simulink model "Model"  (R2023b)
settings: Solver=ode4  StartTime=0.0  StopTime=7.121081656184960e+03  FixedStep=0.1  RelTol=1e-3
values from neighbouring files (symbols this model uses):
  astro_data = astronomicData    [main.m]
  in_cond = initialConditions(astro_data.n_eth)    [main.m]
  orbit_data = orbitData    [main.m]
  pert_data = perturbationData(orbit_data.n_sc)    [main.m]
  sc_data = spaceCraftData    [main.m]
undefined symbols (not defined in the file or in its folder): A_target, k1, k2, Kdx, Kdy, Kdz, Kpx, Kpy, Kpz, sensor_data
libraries: matrix_library x6, simulink x5, vrlib x4
(part 1 of 2)
settings Model: Creator=pierb  LastModifiedBy=pierb

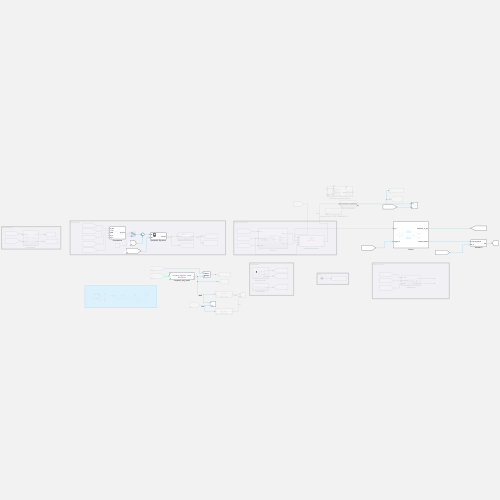
[thumbnail: Simulink's stored preview of the top-level diagram]
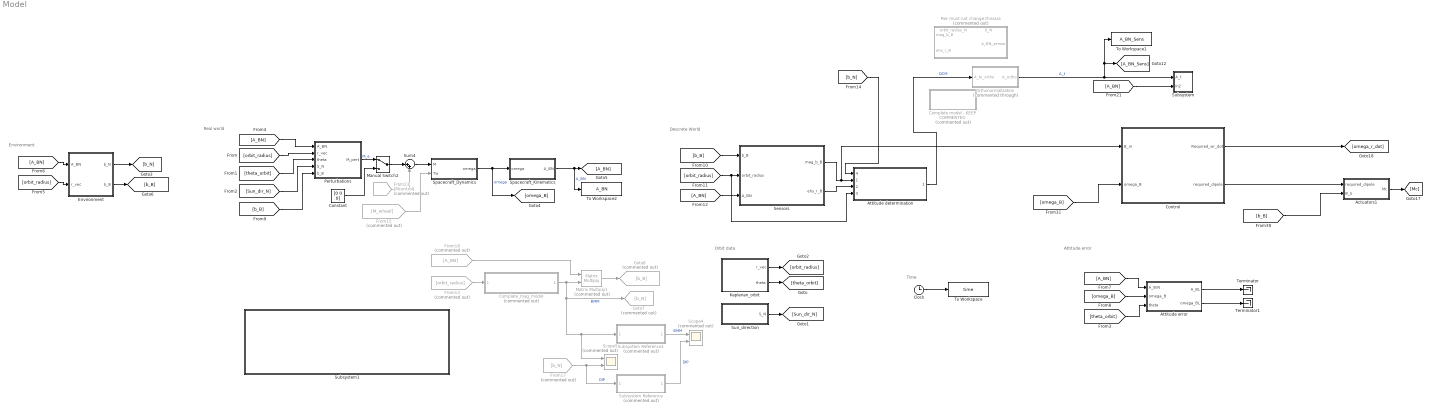
== system Model ==
  note: Descrete World
  note: Environment
  note: Attitude error
  note: Real world
  note: Orbit data
  note: Time
  Actuators1 : Subsystem
  Attitude determination : Subsystem  ReferencedSubsystem=TRIAD
      settings: PortSchema="{\"entries\":[{\"content\":{\"sides\":[{\"content\":{\"connectorIds\":[\"In4\",\"In1\",\"In2\",\"In3\"]},\"type\":\"ConnectorPlacement.EquallySpacedRectSide\",\"uuid\":\"0502630d-a8df-43ec-b57f-23f371792df2\"},{\"content\":{\"connectorIds\":[\"Out1\"],\"side\":\"RIGHT\"},\"type\":\"ConnectorPlacement.EquallySpacedRectSide\",\"uuid\":\"e2538cd4-94c7-4835-89c8-02f932021d19\"},{\"content\":{\"side\":\"TOP\"},\"type\":\"ConnectorPlacement.EquallySpacedRectSide\",\"uuid\":\"052200ab-1f19-47f5-82ad-2a8e946d4726\"},{\"content\":{\"side\":\"BOTTOM\"},\"type\":\"ConnectorPlacement.EquallySpacedRectSide\",\"uuid\":\"8f6caf11-bde2-49b2-b877-be2d81d96931\"}]},\"type\":\"ConnectorPlacement.EquallySpacedConnector\",\"uuid\":\"0adaba7c-309a-4af6-b194-7fbfafdbd17f\"}],\"packageUris\":[\"http://schema.mathworks.com/mf0/Connector/R2020b\"],\"version\":\"1.0\"}"
  Attitude error : Subsystem
  Clock : Clock
  Complete model - KEEP COMMENTED : Subsystem  Commented=on
  Complete_mag_model : Subsystem  Commented=on  ReferencedSubsystem=complete_magnetic_model
  Constant : Constant  Value=[0 0 0]
  Control : Subsystem
  Environment : Subsystem
  From13 : From  Commented=on  GotoTag=orbit_radius
  From15 : From  Commented=on  GotoTag=M_wheel
  From17 : From  Commented=on  GotoTag=b_N
  From18 : From  Commented=on  GotoTag=A_BN
  From23 : From  Commented=on  GotoTag=Mcontrol
  Goto7 : Goto  Commented=on  GotoTag=b_N
  Goto8 : Goto  Commented=on  GotoTag=b_B
  Keplerian_orbit : Subsystem
  Manual Switch2 : ManualSwitch
  Matrix Multiply1 : Product  Commented=on  Multiplication=Matrix(*)
  Orthonormalization : Subsystem  Commented=through
  Perturbations : Subsystem
  Pier must not change thisssss : Subsystem  Commented=on
      settings: PortSchema="{\"entries\":[{\"content\":{\"sides\":[{\"content\":{\"connectorIds\":[\"In1\",\"In2\"]},\"type\":\"ConnectorPlacement.EquallySpacedRectSide\",\"uuid\":\"0502630d-a8df-43ec-b57f-23f371792df2\"},{\"content\":{\"connectorIds\":[\"Out1\"],\"side\":\"RIGHT\"},\"type\":\"ConnectorPlacement.EquallySpacedRectSide\",\"uuid\":\"e2538cd4-94c7-4835-89c8-02f932021d19\"},{\"content\":{\"connectorIds\":[\"In3\",\"In4\"],\"side\":\"TOP\"},\"type\":\"ConnectorPlacement.EquallySpacedRectSide\",\"uuid\":\"052200ab-1f19-47f5-82ad-2a8e946d4726\"}]},\"type\":\"ConnectorPlacement.EquallySpacedConnector\",\"uuid\":\"0adaba7c-309a-4af6-b194-7fbfafdbd17f\"}],\"packageUris\":[\"http://schema.mathworks.com/mf0/Connector/R2020b\"],\"version\":\"1.0\"}"
  Scope4 : Scope  Commented=on  NumInputPorts=2
  Scope5 : Scope  Commented=on  NumInputPorts=2
  Sensors : Subsystem
  Spacecraft_Dynamics : Subsystem
  Spacecraft_Kinematics : Subsystem
  Subsystem : Subsystem
  Subsystem Reference : Subsystem  Commented=on  ReferencedSubsystem=vec_norm
  Subsystem Reference1 : Subsystem  Commented=on  ReferencedSubsystem=vec_norm
  Subsystem1 : Subsystem
  Sum4 : Sum  Inputs=|++
  Sun_direction : Subsystem
  Terminator : Terminator
  Terminator1 : Terminator
  To Workspace : ToWorkspace  VariableName=time  SampleTime=-1
      settings: Save2DSignal=2-D array (concatenate along first dimension)
  To Workspace1 : ToWorkspace  VariableName=A_BN_Sens  SampleTime=-1
  To Workspace2 : ToWorkspace  VariableName=A_BN  SampleTime=-1
  wires:
  Spacecraft_Dynamics/1(omega) -> [omega_B], Spacecraft_Kinematics/1(omega)  "omega"
  Spacecraft_Kinematics/1(A_BN) -> To Workspace2/1, [A_BN]  "A_BN"
  Clock/1 -> To Workspace/1
  Perturbations/1(M_pert) -> Manual Switch2/1  "M_e"
  Manual Switch2/1 -> Sum4/1
  Constant/1 -> Manual Switch2/2
  Attitude error/2(omega_BL) -> Terminator1/1
  Attitude error/1(A_BL) -> Terminator/1
  Keplerian_orbit/2(theta) -> [theta_orbit]
  Sun_direction/1(S_N) -> [Sun_dir_N]
  [orbit_radius] -> Perturbations/2(r_vec)
  [theta_orbit] -> Perturbations/3(theta)
  [Sun_dir_N] -> Perturbations/4(S_N)
  [theta_orbit] -> Attitude error/3(theta)
  [A_BN] -> Perturbations/1(A_BN)
  [A_BN] -> Attitude error/1(A_B/N)
  [omega_B] -> Attitude error/2(omega_B)
  Keplerian_orbit/1(r_vec) -> [orbit_radius]
  [orbit_radius] -> Environment/2(r_vec)
  [A_BN] -> Environment/1(A_BN)
  Environment/2(b_B) -> [b_B]
  Environment/1(b_N) -> [b_N]
  [b_B] -> Perturbations/5(b_B)
  [b_B] -> Sensors/1(b_B)
  [orbit_radius] -> Attitude determination/3, Sensors/2(orbit_radius)
  Sensors/2(ehs_r_B) -> Attitude determination/2
  Attitude determination/1 -> Orthonormalization/1(A_to_ortho)  "DCM"
  [b_N] -> Attitude determination/4
  [A_BN] -> Sensors/3(A_BN)
  Subsystem Reference1/1 -> Scope4/1  "BMM"
  Matrix Multiply1/1 -> Goto8/1
  From18/1 -> Matrix Multiply1/1
  From17/1 -> Subsystem Reference/1, Scope5/2  "DIP"
  Complete_mag_model/1 -> Matrix Multiply1/2, Subsystem Reference1/1, Scope5/1, Goto7/1  "BMM"
  Subsystem Reference/1 -> Scope4/2  "DIP"
  From13/1 -> Complete_mag_model/1
  Sum4/1 -> Spacecraft_Dynamics/1(M)
  From23/1 -> Sum4/2
  From15/1 -> Spacecraft_Dynamics/2(Tw)
  Orthonormalization/1(A_ortho) -> To Workspace1/1, [A_BN_Sens], Subsystem/1(A_t)  "A_t"
  [A_BN] -> Subsystem/2(In2)
  Control/1(Required_wr_dot) -> [omega_r_dot]
  Control/2(required_dipole) -> Actuators1/1(required_dipole)
  [omega_B] -> Control/2(omega_B)
  Actuators1/1(Mc) -> [Mc]
  Sensors/1(mag_b_B) -> Attitude determination/1, Control/1(B_m)
  [b_B] -> Actuators1/2(B_b)

== system Model/Actuators1 ==
  required_dipole : Inport
  B_b : Inport  Port=2
  Apply_inertia : Subsystem
  Cross Product : matrix_library/Cross Product
  Reshape : Reshape  OutputDimensionality=Row vector (2-D)
  Saturation : Saturate  UpperLimit=120  LowerLimit=-120
  Mc : Outport
  wires:
  required_dipole/1 -> Saturation/1
  Saturation/1 -> Cross Product/1
  B_b/1 -> Cross Product/2
  Apply_inertia/1(Torque_omega_dot) -> Mc/1  "I^-1 * M"
  Reshape/1 -> Apply_inertia/1(M)
  Cross Product/1 -> Reshape/1

== system Model/Attitude error ==
  A_B/N : Inport
  omega_B : Inport  Port=2
  theta : Inport  Port=3
  A_LN : Subsystem
  Add : Sum  Inputs=-+
  Constant : Constant  Value=pert_data.w_LN
  Product : Product  Multiplication=Matrix(*)
  Product1 : Product  Multiplication=Matrix(*)
  Reshape : Reshape  OutputDimensionality=Column vector (2-D)
  Reshape1 : Reshape  OutputDimensionality=Column vector (2-D)
  Reshape2 : Reshape  OutputDimensionality=Row vector (2-D)
  To Workspace2 : ToWorkspace  VariableName=w_BL  SampleTime=-1
      settings: Save2DSignal=2-D array (concatenate along first dimension)
  Transpose : Math  Operator=transpose
  A_BL : Outport
  omega_BL : Outport  Port=2
  wires:
  A_LN/1(A_LN) -> Transpose/1
  Transpose/1 -> Product/2
  A_B/N/1 -> Product/1
  Product/1 -> Product1/1, A_BL/1
  omega_B/1 -> Reshape1/1
  Constant/1 -> Reshape/1
  Product1/1 -> Add/1
  Reshape/1 -> Product1/2
  Reshape1/1 -> Add/2
  theta/1 -> A_LN/1(theta)
  Add/1 -> Reshape2/1
  Reshape2/1 -> To Workspace2/1, omega_BL/1

== system Model/Complete model - KEEP COMMENTED ==
  Actuators : Subsystem  Commented=on
  Attitude determination : Subsystem  Commented=on
  Control : Subsystem  Commented=on
  Environment : Subsystem  Commented=on
  Perturbations1 : Subsystem  Commented=on
  Scope1 : Scope  Commented=on
  Sensors : Subsystem  Commented=on
      settings: PortSchema="{\"entries\":[{\"content\":{\"sides\":[{\"content\":{\"connectorIds\":[\"In1\"]},\"type\":\"ConnectorPlacement.EquallySpacedRectSide\",\"uuid\":\"59271294-fd38-4bc9-bb13-2c1f308ccf3d\"},{\"content\":{\"connectorIds\":[\"Out1\"],\"side\":\"RIGHT\"},\"type\":\"ConnectorPlacement.EquallySpacedRectSide\",\"uuid\":\"0ccf848c-1fca-40cd-9aef-56cdc22c78d6\"},{\"content\":{\"connectorIds\":[\"In2\"],\"side\":\"TOP\"},\"type\":\"ConnectorPlacement.EquallySpacedRectSide\",\"uuid\":\"ccb51de9-ba45-4790-8cdc-dbedbef5dfe7\"}]},\"type\":\"ConnectorPlacement.EquallySpacedConnector\",\"uuid\":\"d2012a93-3259-48d9-8262-2c73c3498720\"}],\"packageUris\":[\"http://schema.mathworks.com/mf0/Connector/R2020b\"],\"version\":\"1.0\"}"
  Spacecraft_Dynamics1 : Subsystem  Commented=on
  Spacecraft_Kinematics1 : Subsystem  Commented=on
  Sum : Sum  Commented=on  Inputs=|++
  To Workspace1 : ToWorkspace  Commented=on  VariableName=r_int  SampleTime=-1
      settings: Save2DSignal=2-D array (concatenate along first dimension)
  r_integration : Subsystem  Commented=on
  wires:
  Control/1(Out1) -> Actuators/1(1)
  Actuators/1(Out1) -> Sum/2
  Environment/1(envData) -> Attitude determination/2(envData), Sensors/2(envData)  "envData"
  Perturbations1/1(M_e) -> Sum/1  "M_e"
  Attitude determination/1(A_M) -> Control/1(A_M)  "A_M"
  r_integration/1(r_vec) -> To Workspace1/1, Scope1/1
  Spacecraft_Kinematics1/1(A_T) -> Sensors/1(A_T)  "A_T"
  Sum/1 -> Spacecraft_Dynamics1/1(M)  "M"
  Spacecraft_Dynamics1/1(omega) -> Spacecraft_Kinematics1/1(omega)  "omega"
  Sensors/1(sensorData) -> Attitude determination/1(sensorData)  "sensorData"

== system Model/Control ==
  B_m : Inport
  omega_B : Inport  Port=2
  De-tumbling : Subsystem  TreatAsAtomicUnit=on
  Merge : Merge  Inputs=3  InitialOutput=0
  Merge2 : Merge  Inputs=3  InitialOutput=0
  No control : Subsystem  TreatAsAtomicUnit=on
  Pointing : Subsystem  TreatAsAtomicUnit=on
  String Compare : StringCompare  CaseSensitive=off
  String Compare1 : StringCompare  CaseSensitive=off
  String Constant : StringConstant  String=algorithm
  String Constant1 : StringConstant  String="\"De-tumbling\""
  String Constant2 : StringConstant  String="\"Pointing\""
  XOR : Logic  Operator=NOR  IconShape=distinctive  AllPortsSameDT=off  OutDataTypeStr=boolean
  Required_wr_dot : Outport
  required_dipole : Outport  Port=2
  wires:
  String Constant/1 -> String Compare/2, String Compare1/1
  String Constant1/1 -> String Compare/1
  String Constant2/1 -> String Compare1/2
  String Compare/1 -> De-tumbling/Enable, XOR/1
  String Compare1/1 -> XOR/2, Pointing/Enable
  XOR/1 -> No control/Enable
  De-tumbling/1(Required_wr_dot) -> Merge/1
  No control/1(required_wr_dot) -> Merge/2
  Pointing/1(Required_wr_dot) -> Merge/3
  De-tumbling/2(required_dipole) -> Merge2/1
  No control/2(required_dipole) -> Merge2/2
  Pointing/2(required_dipole) -> Merge2/3
  Merge/1 -> Required_wr_dot/1
  Merge2/1 -> required_dipole/1
  B_m/1 -> De-tumbling/1(B_m)
  omega_B/1 -> De-tumbling/2(omega_B)

== system Model/Environment ==
  A_BN : Inport
  r_vec : Inport  Port=2
  Constant : Constant  Value=astro_data.R_earth
  Constant1 : Constant  Value=pert_data.H0
  Magnetic field : Subsystem  ReferencedSubsystem=dipole_magnetic_model
  Matrix Multiply : Product  Multiplication=Matrix(*)
  Reshape : Reshape  OutputDimensionality=Row vector (2-D)
  Reshape1 : Reshape  OutputDimensionality=Row vector (2-D)
  Subsystem : Subsystem  ReferencedSubsystem=normalize_vec
  Subsystem1 : Subsystem  ReferencedSubsystem=vec_norm
  To Workspace : ToWorkspace  VariableName=env_b_N  SampleTime=-1
      settings: Save2DSignal=2-D array (concatenate along first dimension)
  To Workspace1 : ToWorkspace  VariableName=env_b_B  SampleTime=-1
      settings: Save2DSignal=2-D array (concatenate along first dimension)
  b_N : Outport
  b_B : Outport  Port=2
  wires:
  r_vec/1 -> Subsystem1/1, Subsystem/1
  Reshape/1 -> To Workspace/1
  Reshape1/1 -> To Workspace1/1
  Subsystem/1 -> Magnetic field/1
  Subsystem1/1 -> Magnetic field/2
  Matrix Multiply/1 -> b_B/1, Reshape1/1  "b_B"
  A_BN/1 -> Matrix Multiply/1
  Magnetic field/1 -> Matrix Multiply/2, b_N/1, Reshape/1  "b_N [T]"
  Constant/1 -> Magnetic field/3
  Constant1/1 -> Magnetic field/4

== system Model/Keplerian_orbit ==
  Constant : Constant  Value=in_cond.theta0
  Integrator : Integrator  InitialConditionSource=external  WrapState=on  WrappedStateUpperValue=2*pi  WrappedStateLowerValue=0
  Product : Product
  Reshape : Reshape  OutputDimensionality=Row vector (2-D)
  To Workspace : ToWorkspace  VariableName=kepler_r_vec  SampleTime=-1
      settings: Save2DSignal=2-D array (concatenate along first dimension)
  To Workspace2 : ToWorkspace  VariableName=kepler_theta  SampleTime=-1
      settings: Save2DSignal=2-D array (concatenate along first dimension)
  radius_direction : Subsystem
  radius_mod : Subsystem
  theta_dot : Subsystem
  r_vec : Outport
  theta : Outport  Port=2
  wires:
  theta_dot/1(theta_dot) -> Integrator/1
  Integrator/1 -> theta/1, radius_mod/1(theta), theta_dot/1(theta), radius_direction/1(theta), To Workspace2/1  "theta"
  Constant/1 -> Integrator/2
  radius_direction/1(r_dir) -> Product/1
  radius_mod/1(r_mod) -> Product/2
  Product/1 -> Reshape/1
  Reshape/1 -> To Workspace/1, r_vec/1

== system Model/Orthonormalization ==
  note: $\text{The integration does not preserve the orthonormality of the matrix A, so an iterative method could be implemented. As the error is not high enough to impact substantially the solution, the orthonormalization method is applied only at the first iteration: }\\ A(t) = \frac{3}{2}A_0(t) - \frac{1}{2}A_0(t)A_0^T(t)A_0(t)\\ \text{Note also that this process can be applied only after a certain treshold as been reached to preserve computational power}$
  A_to_ortho : Inport
  Abs : Abs  SaturateOnIntegerOverflow=off
  Constant : Constant  Value=eye(3)
  Constant2 : Constant  Value=1e-6
  If : If  IfExpression=u1 ~= 9
  If Action Subsystem : Subsystem  TreatAsAtomicUnit=on
  If Action Subsystem1 : Subsystem  TreatAsAtomicUnit=on
  Less Than : RelationalOperator  Operator=<=  OutDataTypeStr=boolean  RndMeth=Simplest  InputSameDT=off
  Merge : Merge
  Product1 : Product  Inputs=**  Multiplication=Matrix(*)
  Subtract : Sum  Inputs=+-
  Sum of Elements : Sum  Inputs=+
  Transpose1 : Math  Operator=transpose
  A_ortho : Outport
  wires:
  Product1/1 -> Subtract/1
  Subtract/1 -> Abs/1
  Transpose1/1 -> Product1/2
  Less Than/1 -> Sum of Elements/1
  Constant/1 -> Subtract/2
  Constant2/1 -> Less Than/2
  Abs/1 -> Less Than/1
  Sum of Elements/1 -> If/1
  If/1 -> If Action Subsystem/Action
  If/2 -> If Action Subsystem1/Action
  If Action Subsystem/1(A_ortho) -> Merge/1
  If Action Subsystem1/1(Out1) -> Merge/2
  Merge/1 -> A_ortho/1
  A_to_ortho/1 -> [A_to_ortho]
  [A_to_ortho] -> Product1/1, Transpose1/1
  [A_to_ortho] -> If Action Subsystem1/1(A_to_ortho)
  [A_to_ortho] -> If Action Subsystem/1(A_to_ortho)

== system Model/Perturbations ==
  A_BN : Inport
  r_vec : Inport  Port=2
  theta : Inport  Port=3
  S_N : Inport  Port=4
  b_B : Inport  Port=5
  A_LN : Subsystem
  Add : Sum  Inputs=3
  GG_perturbation : Subsystem  Commented=on
  Magnetic : Subsystem
  SRP : Subsystem  Commented=on
  Subsystem Reference : Subsystem  ReferencedSubsystem=vec_norm
  To Workspace : ToWorkspace  VariableName=perturbations_I_M_GG  SampleTime=-1
      settings: Save2DSignal=2-D array (concatenate along first dimension)
  To Workspace1 : ToWorkspace  VariableName=perturbations_I_M_Mag  SampleTime=-1
      settings: Save2DSignal=2-D array (concatenate along first dimension)
  To Workspace2 : ToWorkspace  VariableName=perturbations_I_M_SRP  SampleTime=-1
      settings: Save2DSignal=2-D array (concatenate along first dimension)
  To Workspace3 : ToWorkspace  VariableName=perturbations_I_M_tot  SampleTime=-1
      settings: Save2DSignal=2-D array (concatenate along first dimension)
  M_pert : Outport
  wires:
  theta/1 -> A_LN/1(theta)
  A_LN/1(A_LN) -> GG_perturbation/1(A_LN)
  A_BN/1 -> SRP/1(A_BN), GG_perturbation/3(A_BN)
  Subsystem Reference/1 -> GG_perturbation/2(r_mod)
  r_vec/1 -> Subsystem Reference/1
  Add/1 -> To Workspace3/1, M_pert/1
  GG_perturbation/1(I_M_GG) -> Add/1, To Workspace/1
  S_N/1 -> SRP/2(S_N)
  Magnetic/1(I_M_Mag) -> To Workspace1/1, Add/3
  SRP/1(I_M_SRP) -> To Workspace2/1, Add/2
  b_B/1 -> Magnetic/1(b_B)

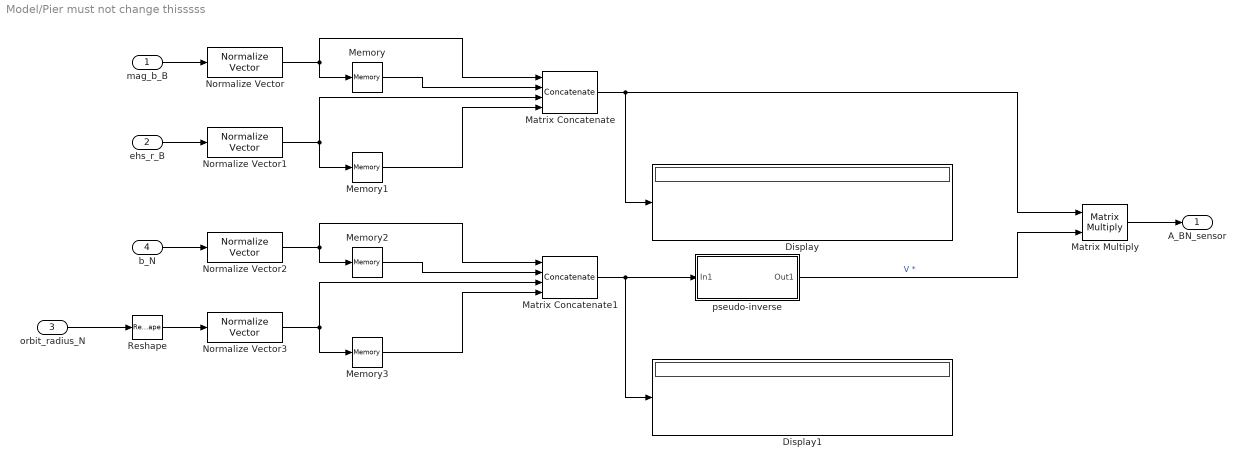
== system Model/Pier must not change thisssss ==
  mag_b_B : Inport
  ehs_r_B : Inport  Port=2
  orbit_radius_N : Inport  Port=3
  b_N : Inport  Port=4
  Display : Display
  Display1 : Display
  Matrix Concatenate : Concatenate  NumInputs=4  Mode=Multidimensional array  ConcatenateDimension=2
  Matrix Concatenate1 : Concatenate  NumInputs=4  Mode=Multidimensional array  ConcatenateDimension=2
  Matrix Multiply : Product  Multiplication=Matrix(*)
  Memory{,1..3} (4 alike) : Memory
  Normalize Vector{,1..3} (4 alike) : vrlib/Utilities/Normalize Vector  maxzero=0
  Reshape : Reshape  OutputDimensionality=Column vector (2-D)
  pseudo-inverse : Subsystem
  A_BN_sensor : Outport
  wires:
  mag_b_B/1 -> Normalize Vector/1
  ehs_r_B/1 -> Normalize Vector1/1
  Matrix Concatenate/1 -> Matrix Multiply/1, Display/1
  Memory/1 -> Matrix Concatenate/2
  Memory1/1 -> Matrix Concatenate/4
  Normalize Vector/1 -> Matrix Concatenate/1, Memory/1
  Normalize Vector1/1 -> Matrix Concatenate/3, Memory1/1
  Normalize Vector2/1 -> Matrix Concatenate1/1, Memory2/1
  Normalize Vector3/1 -> Matrix Concatenate1/3, Memory3/1
  Memory3/1 -> Matrix Concatenate1/4
  b_N/1 -> Normalize Vector2/1
  Memory2/1 -> Matrix Concatenate1/2
  orbit_radius_N/1 -> Reshape/1
  Matrix Concatenate1/1 -> pseudo-inverse/1(In1), Display1/1
  Reshape/1 -> Normalize Vector3/1
  pseudo-inverse/1(Out1) -> Matrix Multiply/2  "V *"
  Matrix Multiply/1 -> A_BN_sensor/1

== system Model/Sensors ==
  b_B : Inport
  orbit_radius : Inport  Port=2
  A_BN : Inport  Port=3
  Digital Clock : DigitalClock  SampleTime=0.1
  Earth horizon sensor : Subsystem  TreatAsAtomicUnit=on  SystemSampleTime=1/sensor_data.magnetometer.freq  ReferencedSubsystem=earth_horizon_sensor
  Magnetometer : Subsystem  SystemSampleTime=1/sensor_data.magnetometer.freq  ReferencedSubsystem=magnetometer_sensor
  Matrix Multiply : Product  Multiplication=Matrix(*)
  Reshape : Reshape  OutputDimensionality=Column vector (2-D)
  Reshape1 : Reshape  OutputDimensionality=Row vector (2-D)
  Reshape2 : Reshape  OutputDimensionality=Row vector (2-D)
  Subsystem Reference : Subsystem  ReferencedSubsystem=normalize_vec
  To Workspace : ToWorkspace  VariableName=sens_magn_B  SampleTime=-1
      settings: Save2DSignal=2-D array (concatenate along first dimension)
  To Workspace1 : ToWorkspace  VariableName=sens_magn_time  SampleTime=-1
      settings: Save2DSignal=2-D array (concatenate along first dimension)
  To Workspace2 : ToWorkspace  VariableName=sens_ehs_r  SampleTime=-1
      settings: Save2DSignal=2-D array (concatenate along first dimension)
  Zero-Order Hold : ZeroOrderHold  SampleTime=1/sensor_data.magnetometer.freq
  Zero-Order Hold1 : ZeroOrderHold  SampleTime=1/sensor_data.horizon.freq
  mag_b_B : Outport
  ehs_r_B : Outport  Port=2
  wires:
  b_B/1 -> Zero-Order Hold/1
  Magnetometer/1 -> mag_b_B/1, Reshape1/1
  Matrix Multiply/1 -> Subsystem Reference/1
  orbit_radius/1 -> Reshape/1
  A_BN/1 -> Matrix Multiply/1
  Reshape/1 -> Matrix Multiply/2
  Reshape1/1 -> To Workspace/1
  Digital Clock/1 -> To Workspace1/1
  Reshape2/1 -> To Workspace2/1
  Earth horizon sensor/1 -> ehs_r_B/1, Reshape2/1
  Zero-Order Hold/1 -> Magnetometer/1
  Zero-Order Hold1/1 -> Earth horizon sensor/1
  Subsystem Reference/1 -> Zero-Order Hold1/1

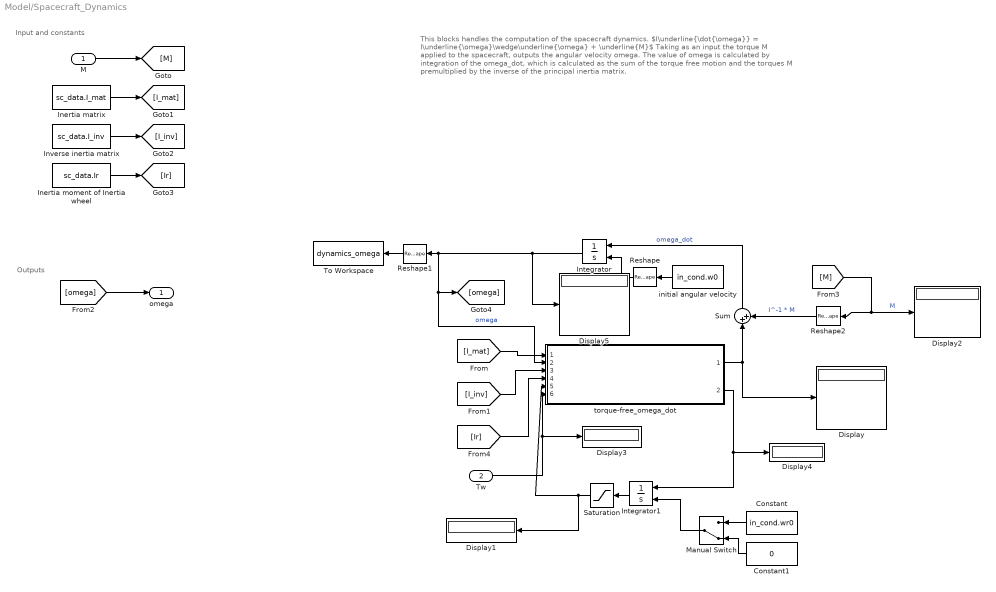
== system Model/Spacecraft_Dynamics ==
  note: This blocks handles the computation of the spacecraft dynamics.
      | $I\underline{\dot{\omega}} = I\underline{\omega}\wedge\underline{\omega} + \underline{M}$
      | Taking as an input the torque M applied to the spacecraft,
      | outputs the angular velocity omega.
      | The value of omega is calculated by integration of the omega_dot, which is calculated as the sum of the torque free motion and the torques M premultiplied by the inverse of the principal inertia matrix.
  note: Outputs
  note: Input and constants
  M : Inport
  Tw : Inport  Port=2
  Constant : Constant  Value=in_cond.wr0
  Constant1 : Constant  Value=0
  Display{,1..5} (6 alike) : Display
  Inertia matrix : Constant  Value=sc_data.I_mat
  Inertia moment of Inertia wheel : Constant  Value=sc_data.Ir
  Integrator : Integrator  InitialConditionSource=external
  Integrator1 : Integrator  InitialConditionSource=external
  Inverse inertia matrix : Constant  Value=sc_data.I_inv
  Manual Switch : ManualSwitch  CurrentSetting=0
  Reshape : Reshape  OutputDimensionality=Column vector (2-D)
  Reshape1 : Reshape  OutputDimensionality=Row vector (2-D)
  Reshape2 : Reshape  OutputDimensionality=Column vector (2-D)
  Saturation : Saturate  UpperLimit=400  LowerLimit=-400
  Sum : Sum  Inputs=|++
  To Workspace : ToWorkspace  VariableName=dynamics_omega  SampleTime=-1
      settings: Save2DSignal=2-D array (concatenate along first dimension)
  initial angular velocity : Constant  Value=in_cond.w0
  torque-free_omega_dot : Subsystem  ReferencedSubsystem=dual_spin_omega_dot
  omega : Outport
  wires:
  [I_mat] -> torque-free_omega_dot/1
  [I_inv] -> torque-free_omega_dot/3
  torque-free_omega_dot/1 -> Display/1, Sum/1
  Integrator/1 -> Display5/1, Reshape1/1, torque-free_omega_dot/2, [omega]  "omega"
  initial angular velocity/1 -> Reshape/1
  Sum/1 -> Integrator/1  "omega_dot"
  [M] -> Reshape2/1, Display2/1  "M"
  Reshape2/1 -> Sum/2  "I^-1 * M"
  Reshape/1 -> Integrator/2
  Reshape1/1 -> To Workspace/1
  Constant1/1 -> Manual Switch/2
  Constant/1 -> Manual Switch/1
  [Ir] -> torque-free_omega_dot/4
  Integrator1/1 -> Saturation/1
  Manual Switch/1 -> Integrator1/2
  Inertia moment of Inertia wheel/1 -> [Ir]
  Inertia matrix/1 -> [I_mat]
  M/1 -> [M]
  [omega] -> omega/1
  Inverse inertia matrix/1 -> [I_inv]
  torque-free_omega_dot/2 -> Integrator1/1, Display4/1
  Tw/1 -> Display3/1, torque-free_omega_dot/6
  Saturation/1 -> torque-free_omega_dot/5, Display1/1

== system Model/Spacecraft_Kinematics ==
  note: This blocks handles the computation of the spacecraft kinematics using the dcm as attitude parameters:
      | $\frac{dA(t)}{dt} = [\omega]\text{^}A(t)$
      | Taking as an input the angular velocity omega, computes the corresponding attitude dcm matrix A(t).
      | As the integration does not preserve the orthonormality of the matrix, an orthonormalization method is implemented.
  omega : Inport
  Gain : Gain  Gain=-1
  Initial condition on dcm attitude : Constant  Value=in_cond.A0
  Integrator : Integrator  InitialConditionSource=external
  Matrix Multiply : Product  Multiplication=Matrix(*)
  Orthonormalization : Subsystem  ReferencedSubsystem=dcm_orthonormalization
  To Workspace : ToWorkspace  VariableName=kinematics_At  SampleTime=-1
  omega_matrix : Subsystem  ReferencedSubsystem=omega_matrix
  A_BN : Outport
  wires:
  Initial condition on dcm attitude/1 -> Integrator/2
  Matrix Multiply/1 -> Integrator/1  "dA/dt"
  Integrator/1 -> Orthonormalization/1  "A_t"
  omega_matrix/1 -> Gain/1  "omega_matrix"
  Gain/1 -> Matrix Multiply/1
  omega/1 -> omega_matrix/1
  Orthonormalization/1 -> To Workspace/1, Matrix Multiply/2, A_BN/1  "A_t"

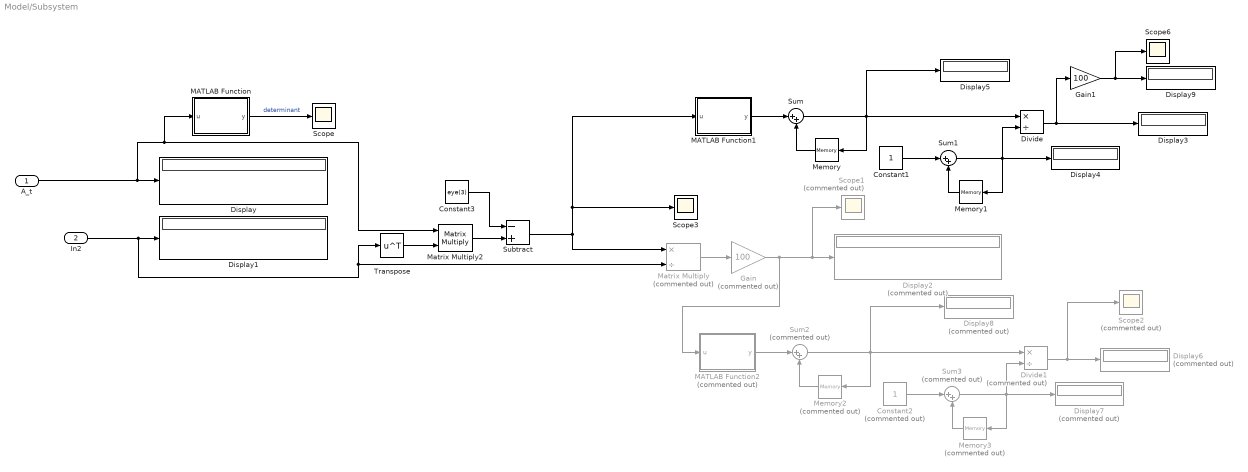
== system Model/Subsystem ==
  A_t : Inport
  In2 : Inport  Port=2
  Constant1 : Constant
  Constant2 : Constant  Commented=on
  Constant3 : Constant  Value=eye(3)
  Display{,1,3..5,9} (6 alike) : Display
  Display{2,6..8} (4 alike) : Display  Commented=on
  Divide : Product  Inputs=*/
  Divide1 : Product  Commented=on  Inputs=*/
  Gain : Gain  Commented=on  Gain=100
  Gain1 : Gain  Gain=100
  MATLAB Function : MATLAB Function  TreatAsAtomicUnit=on
  MATLAB Function1 : MATLAB Function  TreatAsAtomicUnit=on
  MATLAB Function2 : MATLAB Function  Commented=on  TreatAsAtomicUnit=on
  Matrix Multiply : Product  Commented=on  Inputs=*/
  Matrix Multiply2 : Product  Multiplication=Matrix(*)
  Memory : Memory
  Memory1 : Memory
  Memory2 : Memory  Commented=on
  Memory3 : Memory  Commented=on
  Scope : Scope
  Scope1 : Scope  Commented=on
  Scope2 : Scope  Commented=on
  Scope3 : Scope
  Scope6 : Scope
  Subtract : Sum  Inputs=-+
  Sum : Sum  Inputs=|++
  Sum1 : Sum  Inputs=|++
  Sum2 : Sum  Commented=on  Inputs=|++
  Sum3 : Sum  Commented=on  Inputs=|++
  Transpose : Math  Operator=transpose
  wires:
  In2/1 -> Transpose/1, Matrix Multiply/2, Display1/1
  Matrix Multiply/1 -> Gain/1
  Subtract/1 -> Scope3/1, MATLAB Function1/1(u), Matrix Multiply/1
  Divide/1 -> Gain1/1, Display3/1
  Memory2/1 -> Sum2/2
  A_t/1 -> Matrix Multiply2/1, MATLAB Function/1(u), Display/1
  Gain1/1 -> Scope6/1, Display9/1
  Divide1/1 -> Scope2/1, Display6/1
  Gain/1 -> MATLAB Function2/1(u), Display2/1, Scope1/1
  Sum2/1 -> Memory2/1, Divide1/1, Display8/1
  Memory1/1 -> Sum1/2
  MATLAB Function1/1(y) -> Sum/1
  Sum1/1 -> Display4/1, Memory1/1, Divide/2
  Sum/1 -> Display5/1, Divide/1, Memory/1
  Constant1/1 -> Sum1/1
  Memory3/1 -> Sum3/2
  MATLAB Function2/1(y) -> Sum2/1
  Sum3/1 -> Divide1/2, Memory3/1, Display7/1
  Matrix Multiply2/1 -> Subtract/2
  Constant3/1 -> Subtract/1
  Transpose/1 -> Matrix Multiply2/2
  Constant2/1 -> Sum3/1
  MATLAB Function/1(y) -> Scope/1  "determinant"
  Memory/1 -> Sum/2

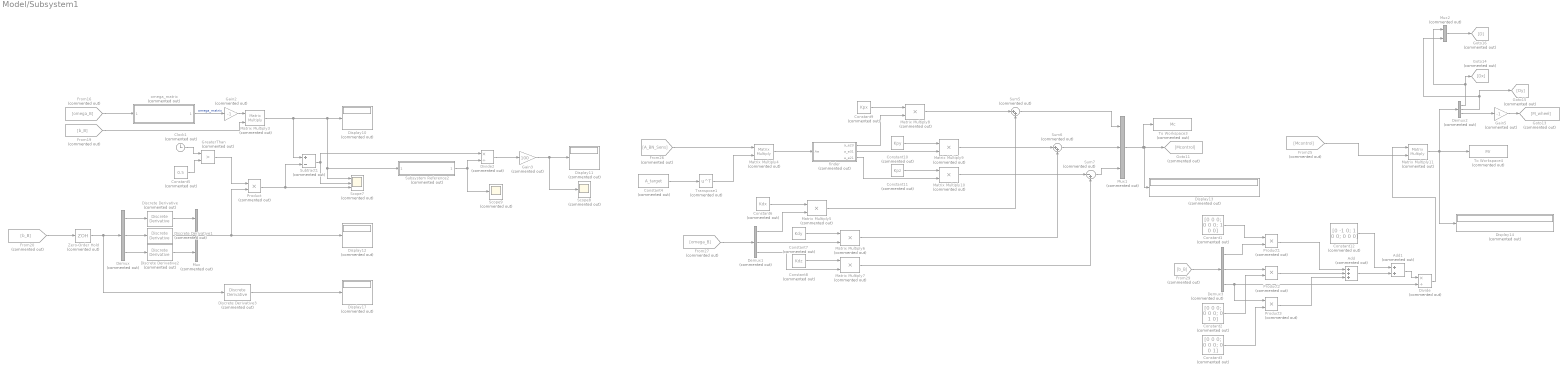
== system Model/Subsystem1 ==
  Add : Sum  Commented=on  Inputs=+++
  Add1 : Sum  Commented=on
  Clock1 : Clock  Commented=on
  Constant1 : Constant  Commented=on  Value=[0 0 0; 0 0 0; 1 0 0]
  Constant10 : Constant  Commented=on  Value=Kpy
  Constant11 : Constant  Commented=on  Value=Kpz
  Constant12 : Constant  Commented=on  Value=[0 -1 0; 1 0 0; 0 0 0]
  Constant2 : Constant  Commented=on  Value=[0 0 0; 0 0 0; 0 1 0]
  Constant3 : Constant  Commented=on  Value=[0 0 0; 0 0 0; 0 0 1]
  Constant4 : Constant  Commented=on  Value=A_target
  Constant5 : Constant  Commented=on  Value=0.5
  Constant6 : Constant  Commented=on  Value=Kdx
  Constant7 : Constant  Commented=on  Value=Kdy
  Constant8 : Constant  Commented=on  Value=Kdz
  Constant9 : Constant  Commented=on  Value=Kpx
  Demux{,1..3} (4 alike) : Demux  Commented=on  Outputs=3
  Discrete Derivative{,1..3} (4 alike) : simulink/Discrete/Discrete Derivative  Commented=on  gainval=1.0  ICPrevScaledInput=0.0  OutMin=[]  OutMax=[]  OutDataType=fixdt(1, 16)  OutScaling=2^-10  DoSatur=off
  Display{10..14,17} (6 alike) : Display  Commented=on
  Divide : Product  Commented=on  Inputs=*/
  Divide2 : Product  Commented=on  Inputs=*/
  From16 : From  Commented=on  GotoTag=omega_B
  From19 : From  Commented=on  GotoTag=b_B
  From20 : From  Commented=on  GotoTag=b_B
  From25 : From  Commented=on  GotoTag=Mcontrol
  From26 : From  Commented=on  GotoTag=A_BN_Sens
  From27 : From  Commented=on  GotoTag=omega_B
  From29 : From  Commented=on  GotoTag=b_B
  Gain2 : Gain  Commented=on  Gain=-1
  Gain3 : Gain  Commented=on  Gain=100
  Gain5 : Gain  Commented=on  Gain=-1
  Goto11 : Goto  Commented=on  GotoTag=Mcontrol
  Goto13 : Goto  Commented=on  GotoTag=M_wheel
  Goto14 : Goto  Commented=on  GotoTag=Dx
  Goto15 : Goto  Commented=on  GotoTag=Dy
  Goto16 : Goto  Commented=on  GotoTag=D
  GreaterThan : RelationalOperator  Commented=on  Operator=>  OutDataTypeStr=boolean  RndMeth=Simplest  InputSameDT=off
  Matrix Multiply{5..10} (6 alike) : Product  Commented=on
  Matrix Multiply11 : Product  Commented=on  Multiplication=Matrix(*)
  Matrix Multiply3 : Product  Commented=on  Multiplication=Matrix(*)
  Matrix Multiply4 : Product  Commented=on  Multiplication=Matrix(*)
  Mux : Mux  Commented=on  Inputs=3
  Mux1 : Mux  Commented=on  Inputs=3
  Mux2 : Mux  Commented=on  Inputs=2
  Product{,1..3} (4 alike) : Product  Commented=on
  Scope7 : Scope  Commented=on  NumInputPorts=3
  Scope8 : Scope  Commented=on
  Scope9 : Scope  Commented=on
  Subsystem Reference2 : Subsystem  Commented=on  ReferencedSubsystem=vec_norm
  Subtract1 : Sum  Commented=on  Inputs=+-
  Sum5 : Sum  Commented=on  Inputs=|++
  Sum6 : Sum  Commented=on  Inputs=|++
  Sum7 : Sum  Commented=on  Inputs=|-+
  To Workspace3 : ToWorkspace  Commented=on  VariableName=Mc  SampleTime=-1
  To Workspace4 : ToWorkspace  Commented=on  VariableName=Mr  SaveFormat=Timeseries  SampleTime=-1
  Transpose1 : Math  Commented=on  Operator=transpose
  Zero-Order Hold : ZeroOrderHold  Commented=on  SampleTime=1/10
  finder : Subsystem  Commented=on
  omega_matrix : Subsystem  Commented=on  ReferencedSubsystem=omega_matrix
  wires:
  Demux2/2 -> Mux2/2, Goto15/1
  From25/1 -> Matrix Multiply11/2
  finder/2(a_e31) -> Matrix Multiply9/2
  Matrix Multiply6/1 -> Sum6/2
  From29/1 -> Demux3/1
  Subtract1/1 -> Scope7/2, Divide2/1
  Discrete Derivative3/1 -> Display17/1
  Demux1/1 -> Matrix Multiply5/2
  Discrete Derivative1/1 -> Mux/2
  Demux3/2 -> Product2/1
  Constant4/1 -> Transpose1/1
  From27/1 -> Demux1/1
  Discrete Derivative/1 -> Mux/1
  Sum6/1 -> Mux1/2
  Gain3/1 -> Scope8/1, Display11/1
  Gain5/1 -> Goto13/1
  Demux1/2 -> Matrix Multiply6/2
  Demux/2 -> Discrete Derivative1/1
  Mux1/1 -> To Workspace3/1, Display13/1, Goto11/1
  Subsystem Reference2/1 -> Divide2/2, Scope9/1
  Sum7/1 -> Mux1/3
  From20/1 -> Zero-Order Hold/1
  Constant5/1 -> GreaterThan/2
  Matrix Multiply11/1 -> Demux2/1, Display14/1, To Workspace4/1
  Product/1 -> Subtract1/2, Scope7/3
  Discrete Derivative2/1 -> Mux/3
  Clock1/1 -> GreaterThan/1
  Matrix Multiply7/1 -> Sum7/2
  From19/1 -> Matrix Multiply3/2
  Product2/1 -> Add/2
  Demux/3 -> Discrete Derivative2/1
  Zero-Order Hold/1 -> Discrete Derivative3/1, Demux/1
  Product3/1 -> Add/3
  Demux2/1 -> Mux2/1, Goto14/1
  Constant7/1 -> Matrix Multiply6/1
  Add/1 -> Add1/2
  Divide2/1 -> Gain3/1
  Mux/1 -> Display12/1, Product/2
  Matrix Multiply4/1 -> finder/1(Ae)
  Matrix Multiply5/1 -> Sum5/2
  omega_matrix/1 -> Gain2/1  "omega_matrix"
  Matrix Multiply3/1 -> Subtract1/1, Scope7/1, Subsystem Reference2/1, Display10/1
  Gain2/1 -> Matrix Multiply3/1
  Matrix Multiply8/1 -> Sum5/1
  From16/1 -> omega_matrix/1
  finder/1(a_e23) -> Matrix Multiply8/2
  Constant10/1 -> Matrix Multiply9/1
  Constant1/1 -> Product1/1
  Demux1/3 -> Matrix Multiply7/2
  From26/1 -> Matrix Multiply4/1
  Demux2/3 -> Gain5/1
  Constant9/1 -> Matrix Multiply8/1
  Constant12/1 -> Add1/1
  Matrix Multiply10/1 -> Sum7/1
  Sum5/1 -> Mux1/1
  Demux3/1 -> Product1/2
  Constant8/1 -> Matrix Multiply7/1
  GreaterThan/1 -> Product/1
  Constant2/1 -> Product2/2
  Demux3/3 -> Divide/2, Product3/1
  Mux2/1 -> Goto16/1
  Constant3/1 -> Product3/2
  Constant6/1 -> Matrix Multiply5/1
  Constant11/1 -> Matrix Multiply10/1
  Matrix Multiply9/1 -> Sum6/1
  Divide/1 -> Matrix Multiply11/1
  Add1/1 -> Divide/1
  Product1/1 -> Add/1
  finder/3(a_e21) -> Matrix Multiply10/2
  Demux/1 -> Discrete Derivative/1
  Transpose1/1 -> Matrix Multiply4/2

== system Model/Sun_direction ==
  Clock : Clock
  Cos : Trigonometry  Operator=cos
  Gain : Gain  Gain=astro_data.n_sun
  Gain1 : Gain  Gain=astro_data.R_sun
  Gain2 : Gain  Gain=cos(astro_data.eps)
  Gain3 : Gain  Gain=sin(astro_data.eps)
  Reshape : Reshape  OutputDimensionality=Column vector (2-D)
  Sin : Trigonometry
  Vector Concatenate : Concatenate  NumInputs=3
  S_N : Outport
  wires:
  Clock/1 -> Gain/1
  Vector Concatenate/1 -> Gain1/1
  Gain1/1 -> Reshape/1
  Gain/1 -> Cos/1, Sin/1
  Cos/1 -> Vector Concatenate/1
  Sin/1 -> Gain2/1, Gain3/1
  Gain2/1 -> Vector Concatenate/2
  Gain3/1 -> Vector Concatenate/3
  Reshape/1 -> S_N/1

== system Model/Actuators1/Apply_inertia ==
  M : Inport
  Constant : Constant  Value=sc_data.I_inv
  Matrix Multiply : Product  Multiplication=Matrix(*)
  Reshape : Reshape  OutputDimensionality=Column vector (2-D)
  Reshape1 : Reshape  OutputDimensionality=Row vector (2-D)
  Torque_omega_dot : Outport
  wires:
  M/1 -> Reshape/1
  Matrix Multiply/1 -> Reshape1/1
  Reshape/1 -> Matrix Multiply/2
  Reshape1/1 -> Torque_omega_dot/1
  Constant/1 -> Matrix Multiply/1

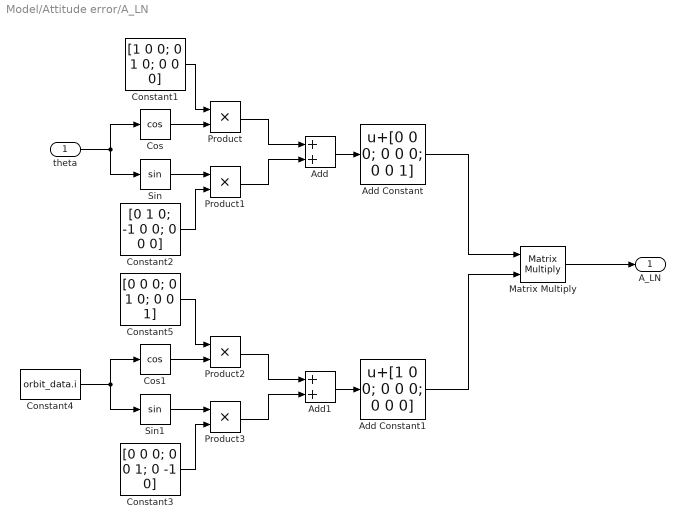
== system Model/Attitude error/A_LN ==
  theta : Inport
  Add : Sum
  Add Constant : Bias  Bias=[0 0 0; 0 0 0; 0 0 1]  SaturateOnIntegerOverflow=off
  Add Constant1 : Bias  Bias=[1 0 0; 0 0 0; 0 0 0]  SaturateOnIntegerOverflow=off
  Add1 : Sum
  Constant1 : Constant  Value=[1 0 0; 0 1 0; 0 0 0]
  Constant2 : Constant  Value=[0 1 0; -1 0 0; 0 0 0]
  Constant3 : Constant  Value=[0 0 0; 0 0 1; 0 -1 0]
  Constant4 : Constant  Value=orbit_data.i
  Constant5 : Constant  Value=[0 0 0; 0 1 0; 0 0 1]
  Cos : Trigonometry  Operator=cos
  Cos1 : Trigonometry  Operator=cos
  Matrix Multiply : Product  Multiplication=Matrix(*)
  Product{,1..3} (4 alike) : Product
  Sin : Trigonometry
  Sin1 : Trigonometry
  A_LN : Outport
  wires:
  Matrix Multiply/1 -> A_LN/1
  theta/1 -> Sin/1, Cos/1
  Constant1/1 -> Product/1
  Cos/1 -> Product/2
  Sin/1 -> Product1/1
  Constant2/1 -> Product1/2
  Product/1 -> Add/1
  Product1/1 -> Add/2
  Add/1 -> Add Constant/1
  Add1/1 -> Add Constant1/1
  Product3/1 -> Add1/2
  Product2/1 -> Add1/1
  Constant3/1 -> Product3/2
  Sin1/1 -> Product3/1
  Cos1/1 -> Product2/2
  Constant5/1 -> Product2/1
  Constant4/1 -> Cos1/1, Sin1/1
  Add Constant1/1 -> Matrix Multiply/2
  Add Constant/1 -> Matrix Multiply/1

== system Model/Complete model - KEEP COMMENTED/Actuators ==
  1 : Inport
  Out1 : Outport
  wires:
  1/1 -> Out1/1

== system Model/Complete model - KEEP COMMENTED/Attitude determination ==
  sensorData : Inport
  envData : Inport  Port=2
  A_M : Outport
  wires:
  sensorData/1 -> A_M/1

== system Model/Complete model - KEEP COMMENTED/Control ==
  A_M : Inport
  Out1 : Outport
  wires:
  A_M/1 -> Out1/1

== system Model/Complete model - KEEP COMMENTED/Environment ==
  envData : Outport
  wires:
  ? -> envData/1

== system Model/Complete model - KEEP COMMENTED/Perturbations1 ==
  M_e : Outport
  wires:
  ? -> M_e/1

== system Model/Complete model - KEEP COMMENTED/Sensors ==
  A_T : Inport
  envData : Inport  Port=2
  sensorData : Outport
  wires:
  A_T/1 -> sensorData/1

== system Model/Complete model - KEEP COMMENTED/Spacecraft_Dynamics1 ==
  note: This blocks handles the computation of the spacecraft dynamics.
      | Taking as an input the torque M applied to the spacecraft,
      | outputs the angular velocity omega.
      | The value of omega is calculated by integration of the omega_dot, which is calculated as the sum of the torque free motion and the torques M premultiplied by the inverse of the principal inertia matrix.
  M : Inport
  Apply_inertia : Subsystem
  Inertia matrix : Constant  Value=sc_data.I_mat
  Integrator : Integrator  InitialConditionSource=external
  Inverse inertia matrix : Constant  Value=sc_data.I_inv
  Sum : Sum  Inputs=|++
  initial angular velocity : Constant  Value=in_cond.w0
  torque-free_omega_dot : Subsystem
  omega : Outport
  wires:
  [I_inv] -> Apply_inertia/2(I_inv)
  Apply_inertia/1(Torque_omega_dot) -> Sum/2  "I^-1 * M"
  [M] -> Apply_inertia/1(M)  "M"
  Sum/1 -> Integrator/1  "omega_dot"
  initial angular velocity/1 -> Integrator/2
  Integrator/1 -> torque-free_omega_dot/2(omega), [omega]  "omega"
  torque-free_omega_dot/1(torque-free_omega_dot) -> Sum/1
  [I_inv] -> torque-free_omega_dot/3(Inverse Inertia)
  [I_mat] -> torque-free_omega_dot/1(Inertia matrix)
  [omega] -> omega/1
  Inverse inertia matrix/1 -> [I_inv]
  Inertia matrix/1 -> [I_mat]
  M/1 -> [M]

== system Model/Complete model - KEEP COMMENTED/Spacecraft_Kinematics1 ==
  note: This blocks handles the computation of the spacecraft kinematics using the dcm as attitude parameters:
      | $\frac{dA(t)}{dt} = [\omega]\text{^}A(t)$
      | Taking as an input the angular velocity omega, computes the corresponding attitude dcm matrix A(t).
      | As the integration does not preserve the orthonormality of the matrix, an orthonormalization method is implemented.
  omega : Inport
  Gain : Gain  Gain=-1
  Initial condition on dcm attitude : Constant  Value=in_cond.A0
  Integrator : Integrator  InitialConditionSource=external
  Matrix Multiply : Product  Multiplication=Matrix(*)
  Orthonormalization : Subsystem
  To Workspace : ToWorkspace  VariableName=At  SampleTime=-1
  omega_matrix : Subsystem
  A_T : Outport
  wires:
  Orthonormalization/1(A_ortho) -> A_T/1, Matrix Multiply/2, To Workspace/1  "A_t"
  omega/1 -> omega_matrix/1(omega)
  Gain/1 -> Matrix Multiply/1
  omega_matrix/1(omega_matrix) -> Gain/1  "omega_matrix"
  Integrator/1 -> Orthonormalization/1(A_to_ortho)  "A_t"
  Matrix Multiply/1 -> Integrator/1  "dA/dt"
  Initial condition on dcm attitude/1 -> Integrator/2

== system Model/Complete model - KEEP COMMENTED/r_integration ==
  Constant : Constant  Value="[0    9.4702    5.4676]"
  Constant1 : Constant  Value=[5000 0 0]
  Constant2 : Constant  Value=3
  Divide : Product  Inputs=*/
  Gain : Gain  Gain=-astro_data.muE
  Integrator : Integrator  InitialConditionSource=external
  Integrator1 : Integrator  InitialConditionSource=external
  Math Function : Math  Operator=pow
  Subsystem : Subsystem
  r_vec : Outport
  wires:
  Integrator/1 -> Integrator1/1
  Constant/1 -> Integrator/2
  Constant1/1 -> Integrator1/2
  Integrator1/1 -> r_vec/1, Subsystem/1(Vector), Gain/1
  Gain/1 -> Divide/1
  Subsystem/1(Norm) -> Math Function/1
  Math Function/1 -> Divide/2
  Constant2/1 -> Math Function/2
  Divide/1 -> Integrator/1

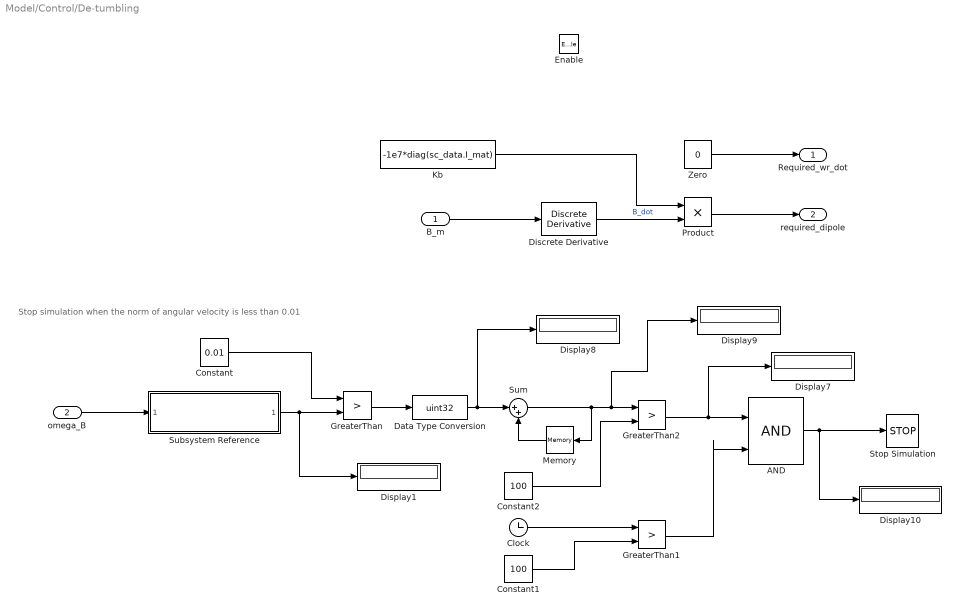
== system Model/Control/De-tumbling ==
  note: Stop simulation when the norm of angular velocity is less than 0.01
  B_m : Inport
  omega_B : Inport  Port=2
  Enable : EnablePort
  AND : Logic  IconShape=distinctive  AllPortsSameDT=off  OutDataTypeStr=boolean
  Clock : Clock
  Constant : Constant  Value=0.01
  Constant1 : Constant  Value=100
  Constant2 : Constant  Value=100
  Data Type Conversion : DataTypeConversion  OutDataTypeStr=uint32  SaturateOnIntegerOverflow=off  RndMeth=Floor
  Discrete Derivative : simulink/Discrete/Discrete Derivative  gainval=1.0  ICPrevScaledInput=0.0  OutMin=[]  OutMax=[]  OutDataType=fixdt(1, 16)  OutScaling=2^-10  DoSatur=off
  Display{1,7..10} (5 alike) : Display
  GreaterThan : RelationalOperator  Operator=>  OutDataTypeStr=boolean  RndMeth=Simplest  InputSameDT=off
  GreaterThan1 : RelationalOperator  Operator=>  OutDataTypeStr=boolean  RndMeth=Simplest  InputSameDT=off
  GreaterThan2 : RelationalOperator  Operator=>  OutDataTypeStr=boolean  RndMeth=Simplest  InputSameDT=off
  Kb : Constant  Value=-1e7*diag(sc_data.I_mat)
  Memory : Memory
  Product : Product
  Stop Simulation : Stop
  Subsystem Reference : Subsystem  ReferencedSubsystem=vec_norm
  Sum : Sum  Inputs=|++
  Zero : Constant  Value=0  OutDataTypeStr=Inherit: Inherit via back propagation
  Required_wr_dot : Outport
  required_dipole : Outport  Port=2
  wires:
  Sum/1 -> Display9/1, GreaterThan2/1, Memory/1
  GreaterThan2/1 -> Display7/1, AND/1
  Constant1/1 -> GreaterThan1/2
  Kb/1 -> Product/1
  AND/1 -> Stop Simulation/1, Display10/1
  Constant/1 -> GreaterThan/1
  B_m/1 -> Discrete Derivative/1
  omega_B/1 -> Subsystem Reference/1
  Subsystem Reference/1 -> Display1/1, GreaterThan/2
  Memory/1 -> Sum/2
  GreaterThan1/1 -> AND/2
  Data Type Conversion/1 -> Display8/1, Sum/1
  Discrete Derivative/1 -> Product/2  "B_dot"
  Zero/1 -> Required_wr_dot/1
  Clock/1 -> GreaterThan1/1
  Product/1 -> required_dipole/1
  GreaterThan/1 -> Data Type Conversion/1
  Constant2/1 -> GreaterThan2/2

== system Model/Control/No control ==
  Enable : EnablePort
  Constant : Constant  Value=0
  Constant1 : Constant  Value=zeros(3, 1)
  required_wr_dot : Outport
  required_dipole : Outport  Port=2
  wires:
  Constant/1 -> required_wr_dot/1
  Constant1/1 -> required_dipole/1

== system Model/Control/Pointing ==
  omega_b : Inport
  omega_err : Inport  Port=2
  DCM : Inport  Port=3
  A_target : Inport  Port=4
  Enable : EnablePort
  Constant : Constant  Value=0
  Constant1 : Constant  Value=zeros(3,1)
  Lyapunov function : Subsystem
  Required_wr_dot : Outport
  required_dipole : Outport  Port=2
  wires:
  Constant/1 -> Required_wr_dot/1
  Constant1/1 -> required_dipole/1
  omega_b/1 -> Lyapunov function/1(omega_b)
  A_target/1 -> Lyapunov function/4(A_target)
  DCM/1 -> Lyapunov function/3(DCM)
  omega_err/1 -> Lyapunov function/2(omega_err)

== system Model/Keplerian_orbit/radius_direction ==
  theta : Inport
  Cos : Trigonometry  Operator=cos
  Cos1 : Trigonometry
  Gain : Gain  Gain=cos(orbit_data.i)
  Gain2 : Gain  Gain=sin(orbit_data.i)
  Vector Concatenate : Concatenate  NumInputs=3
  r_dir : Outport
  wires:
  Vector Concatenate/1 -> r_dir/1
  Cos/1 -> Vector Concatenate/1
  theta/1 -> Cos1/1, Cos/1
  Gain/1 -> Vector Concatenate/2
  Cos1/1 -> Gain2/1, Gain/1
  Gain2/1 -> Vector Concatenate/3

== system Model/Keplerian_orbit/radius_mod ==
  theta : Inport
  Add Constant : Bias  Bias=1  SaturateOnIntegerOverflow=off
  Constant : Constant  Value=orbit_data.a*(1-orbit_data.e^2)
  Cos : Trigonometry  Operator=cos
  Divide : Product  Inputs=*/
  Gain : Gain  Gain=orbit_data.e
  r_mod : Outport
  wires:
  Constant/1 -> Divide/1
  Divide/1 -> r_mod/1
  theta/1 -> Cos/1
  Cos/1 -> Gain/1
  Gain/1 -> Add Constant/1
  Add Constant/1 -> Divide/2

== system Model/Keplerian_orbit/theta_dot ==
  theta : Inport
  Add Constant : Bias  Bias=1  SaturateOnIntegerOverflow=off
  Constant : Constant  Value=orbit_data.e^2
  Constant1 : Constant
  Constant2 : Constant  Value=3/2
  Constant3 : Constant  Value=orbit_data.n_sc
  Cos : Trigonometry  Operator=cos
  Divide : Product  Inputs=**/
  Gain : Gain  Gain=orbit_data.e
  Power : Math  Operator=pow
  Power1 : Math  Operator=square
  Subtract : Sum  Inputs=+-
  theta_dot : Outport
  wires:
  Divide/1 -> theta_dot/1
  Power/1 -> Divide/3
  Constant/1 -> Subtract/2
  Constant1/1 -> Subtract/1
  Subtract/1 -> Power/1
  Constant2/1 -> Power/2
  theta/1 -> Cos/1
  Cos/1 -> Gain/1
  Gain/1 -> Add Constant/1
  Add Constant/1 -> Power1/1
  Power1/1 -> Divide/2
  Constant3/1 -> Divide/1

== system Model/Orthonormalization/If Action Subsystem ==
  A_to_ortho : Inport
  Action Port : ActionPort  ActionPortLabel=if(u1 ~= 9)
  Add : Sum  Inputs=+-
  Gain : Gain  Gain=3/2
  Gain1 : Gain  Gain=1/2
  Product : Product  Inputs=***  Multiplication=Matrix(*)
  Transpose : Math  Operator=transpose
  A_ortho : Outport
  wires:
  Gain/1 -> Add/1
  Gain1/1 -> Add/2
  Transpose/1 -> Product/2
  A_to_ortho/1 -> Product/3, Transpose/1, Product/1, Gain/1
  Product/1 -> Gain1/1
  Add/1 -> A_ortho/1

== system Model/Orthonormalization/If Action Subsystem1 ==
  A_to_ortho : Inport
  Action Port : ActionPort  ActionPortLabel=else
  Out1 : Outport
  wires:
  A_to_ortho/1 -> Out1/1

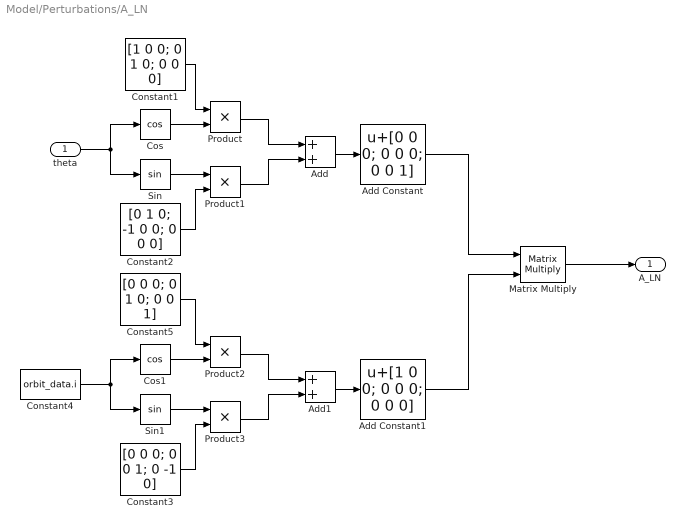
== system Model/Perturbations/A_LN ==
  theta : Inport
  Add : Sum
  Add Constant : Bias  Bias=[0 0 0; 0 0 0; 0 0 1]  SaturateOnIntegerOverflow=off
  Add Constant1 : Bias  Bias=[1 0 0; 0 0 0; 0 0 0]  SaturateOnIntegerOverflow=off
  Add1 : Sum
  Constant1 : Constant  Value=[1 0 0; 0 1 0; 0 0 0]
  Constant2 : Constant  Value=[0 1 0; -1 0 0; 0 0 0]
  Constant3 : Constant  Value=[0 0 0; 0 0 1; 0 -1 0]
  Constant4 : Constant  Value=orbit_data.i
  Constant5 : Constant  Value=[0 0 0; 0 1 0; 0 0 1]
  Cos : Trigonometry  Operator=cos
  Cos1 : Trigonometry  Operator=cos
  Matrix Multiply : Product  Multiplication=Matrix(*)
  Product{,1..3} (4 alike) : Product
  Sin : Trigonometry
  Sin1 : Trigonometry
  A_LN : Outport
  wires:
  Matrix Multiply/1 -> A_LN/1
  theta/1 -> Sin/1, Cos/1
  Constant1/1 -> Product/1
  Cos/1 -> Product/2
  Sin/1 -> Product1/1
  Constant2/1 -> Product1/2
  Product/1 -> Add/1
  Product1/1 -> Add/2
  Add/1 -> Add Constant/1
  Add1/1 -> Add Constant1/1
  Product3/1 -> Add1/2
  Product2/1 -> Add1/1
  Constant3/1 -> Product3/2
  Sin1/1 -> Product3/1
  Cos1/1 -> Product2/2
  Constant5/1 -> Product2/1
  Constant4/1 -> Cos1/1, Sin1/1
  Add Constant1/1 -> Matrix Multiply/2
  Add Constant/1 -> Matrix Multiply/1

== system Model/Perturbations/GG_perturbation ==
  A_LN : Inport
  r_mod : Inport  Port=2
  A_BN : Inport  Port=3
  Constant : Constant  Value=[1; 0; 0]
  Constant1 : Constant  Value=astro_data.muE
  Constant2 : Constant  Value=3
  Constant3 : Constant  Value=sc_data.I_mat
  Constant4 : Constant  Value=sc_data.I_inv
  Divide : Product  Inputs=*/
  Gain : Gain  Gain=-3
  Matrix Multiply : Product  Multiplication=Matrix(*)
  Matrix Multiply1 : Product  Multiplication=Matrix(*)
  Power : Math  Operator=pow
  Product : Product
  Reshape : Reshape  OutputDimensionality=Row vector (2-D)
  Subsystem : Subsystem
  Transpose : Math  Operator=transpose
  I_M_GG : Outport
  wires:
  A_BN/1 -> Matrix Multiply/1
  A_LN/1 -> Transpose/1
  Transpose/1 -> Matrix Multiply/2
  Matrix Multiply/1 -> Matrix Multiply1/1  "A_BL"
  Constant/1 -> Matrix Multiply1/2
  Product/1 -> Gain/1
  Gain/1 -> Reshape/1
  Constant1/1 -> Divide/1
  r_mod/1 -> Power/1
  Power/1 -> Divide/2
  Constant2/1 -> Power/2
  Divide/1 -> Product/2
  Reshape/1 -> I_M_GG/1
  Matrix Multiply1/1 -> Subsystem/2(c1 c2 c3)  "[c1 c2 c3]"
  Subsystem/1(M_GG_vec) -> Product/1
  Constant3/1 -> Subsystem/1(Inertia matrix)
  Constant4/1 -> Subsystem/3(Inverse Inertia)

== system Model/Perturbations/Magnetic ==
  b_B : Inport
  Apply_inertia : Subsystem
  Constant3 : Constant  Value=[0.01 0.05 0.01]'
  Cross Product : matrix_library/Cross Product
  Reshape1 : Reshape  OutputDimensionality=Row vector (2-D)
  To Workspace1 : ToWorkspace  VariableName=perturbations_M_Mag  SampleTime=-1
      settings: Save2DSignal=2-D array (concatenate along first dimension)
  I_M_Mag : Outport
  wires:
  b_B/1 -> Cross Product/2  "b_B"
  Cross Product/1 -> Reshape1/1  "M_Mag"
  Constant3/1 -> Cross Product/1
  Reshape1/1 -> To Workspace1/1, Apply_inertia/1(M)  "M_mag"
  Apply_inertia/1(Torque_omega_dot) -> I_M_Mag/1  "I^-1 * M"

== system Model/Perturbations/SRP ==
  A_BN : Inport
  S_N : Inport  Port=2
  Apply_inertia : Subsystem
  Constant : Constant  Value=sc_data.NB
  Constant1 : Constant  Value=sc_data.rhoS
  Constant2 : Constant  Value=sc_data.rhoD
  Constant3 : Constant  Value=sc_data.A
  Constant4 : Constant  Value=sc_data.rF
  Divide : Product  Inputs=*/
  For Each Subsystem : Subsystem  TreatAsAtomicUnit=on
  Matrix Multiply : Product  Multiplication=Matrix(*)
  Norm : Subsystem
  Scope : Scope
  Sum of Elements : Sum  Inputs=+  CollapseMode=Specified dimension
  To Workspace1 : ToWorkspace  VariableName=perturbations_M_SRP  SampleTime=-1
      settings: Save2DSignal=2-D array (concatenate along first dimension)
  I_M_SRP : Outport
  wires:
  A_BN/1 -> Matrix Multiply/1
  S_N/1 -> Matrix Multiply/2
  Matrix Multiply/1 -> Norm/1(In1), Divide/1  "S_B"
  Constant2/1 -> For Each Subsystem/3(rhoD_i)
  Constant1/1 -> For Each Subsystem/2(rhoS_i)
  Constant/1 -> For Each Subsystem/1(NB_i)
  Constant3/1 -> For Each Subsystem/4(A_i)
  Divide/1 -> For Each Subsystem/6(SB)
  Norm/1(Out1) -> Divide/2
  For Each Subsystem/1(Mi) -> Sum of Elements/1
  Constant4/1 -> For Each Subsystem/5(rF_i)
  Sum of Elements/1 -> Scope/1, To Workspace1/1, Apply_inertia/1(M)  "M_SRP"
  Apply_inertia/1(Torque_omega_dot) -> I_M_SRP/1  "I^-1 * M"

== system Model/Pier must not change thisssss/pseudo-inverse ==
  In1 : Inport
  Product : Product  Multiplication=Matrix(*)
  Product1 : Product  Inputs=*/  Multiplication=Matrix(*)
  Transpose1 : Math  Operator=transpose
  Out1 : Outport
  wires:
  Product1/1 -> Out1/1
  In1/1 -> Product/1, Transpose1/1
  Transpose1/1 -> Product/2, Product1/1
  Product/1 -> Product1/2

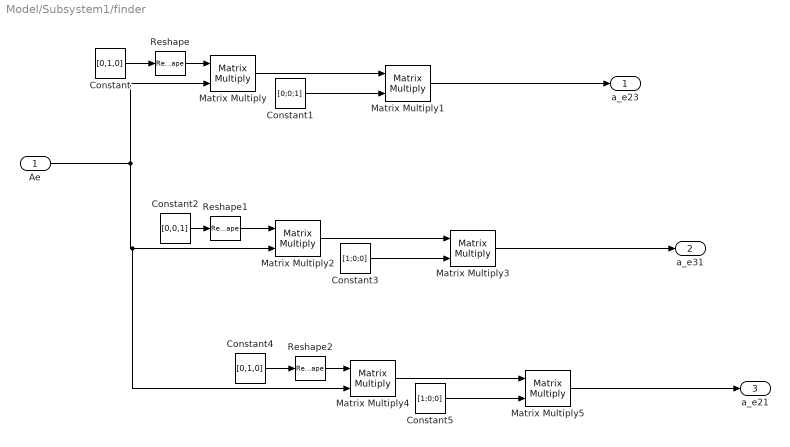
== system Model/Subsystem1/finder ==
  Ae : Inport
  Constant : Constant  Value=[0,1,0]
  Constant1 : Constant  Value=[0;0;1]
  Constant2 : Constant  Value=[0,0,1]
  Constant3 : Constant  Value=[1;0;0]
  Constant4 : Constant  Value=[0,1,0]
  Constant5 : Constant  Value=[1;0;0]
  Matrix Multiply{,1..5} (6 alike) : Product  Multiplication=Matrix(*)
  Reshape : Reshape  OutputDimensionality=Row vector (2-D)
  Reshape1 : Reshape  OutputDimensionality=Row vector (2-D)
  Reshape2 : Reshape  OutputDimensionality=Row vector (2-D)
  a_e23 : Outport
  a_e31 : Outport  Port=2
  a_e21 : Outport  Port=3
  wires:
  Matrix Multiply/1 -> Matrix Multiply1/1
  Constant1/1 -> Matrix Multiply1/2
  Matrix Multiply1/1 -> a_e23/1
  Constant2/1 -> Reshape1/1
  Matrix Multiply2/1 -> Matrix Multiply3/1
  Constant3/1 -> Matrix Multiply3/2
  Matrix Multiply3/1 -> a_e31/1
  Ae/1 -> Matrix Multiply4/2, Matrix Multiply2/2, Matrix Multiply/2
  Constant4/1 -> Reshape2/1
  Matrix Multiply4/1 -> Matrix Multiply5/1
  Constant5/1 -> Matrix Multiply5/2
  Matrix Multiply5/1 -> a_e21/1
  Constant/1 -> Reshape/1
  Reshape/1 -> Matrix Multiply/1
  Reshape1/1 -> Matrix Multiply2/1
  Reshape2/1 -> Matrix Multiply4/1

== system Model/Complete model - KEEP COMMENTED/Spacecraft_Dynamics1/Apply_inertia ==
  M : Inport
  I_inv : Inport  Port=2
  Matrix Multiply : Product  Multiplication=Matrix(*)
  Torque_omega_dot : Outport
  wires:
  Matrix Multiply/1 -> Torque_omega_dot/1
  I_inv/1 -> Matrix Multiply/1
  M/1 -> Matrix Multiply/2

== system Model/Complete model - KEEP COMMENTED/Spacecraft_Dynamics1/torque-free_omega_dot ==
  Inertia matrix : Inport
  omega : Inport  Port=2
  Inverse Inertia : Inport  Port=3
  Cross Product : matrix_library/Cross Product
  Matrix Divide : Product  Inputs=**  Multiplication=Matrix(*)
  Product : Product  Multiplication=Matrix(*)
  torque-free_omega_dot : Outport
  wires:
  Cross Product/1 -> Matrix Divide/2  "h_cross_om"
  omega/1 -> Product/2, Cross Product/2  "omega"
  Inertia matrix/1 -> Product/1  "I_matrix"
  Inverse Inertia/1 -> Matrix Divide/1
  Product/1 -> Cross Product/1  "h"
  Matrix Divide/1 -> torque-free_omega_dot/1
